simulink model "play"  (R2024a)
settings: Solver=ode1  StartTime=0.0  StopTime=inf  FixedStep=1/10  RelTol=1e-3  EnableMultiTasking=on
undefined symbols (not defined in the file): HIL, Host
libraries: quarc_library x8, simulink_extras x1, simulink x1
settings Model: Creator=msaravanan  LastModifiedBy=msaravanan
settings SolverCC: PositivePriorityOrder=on
settings RTWCC: Description=QUARC Win64 Target Using Toolchain  SystemTargetFile=quarc_win64.tlc  Toolchain=QUARC win64 | nmake (64-bit Windows)  BuildConfiguration=Faster Runs
settings STFCustomTargetCC: ConcurrentExecutionCompliant=on  SystemTargetFile=quarc_win64.tlc
settings GRTTargetCC: ParMdlRefBuildCompliant=off  CompOptLevelCompliant=off  CombineOutputUpdateFcns=off  MatFileLogging=off  CPPClassGenCompliant=off  GRTInterface=on  ExtMode=on  ExtModeMexFile=quarc_comm

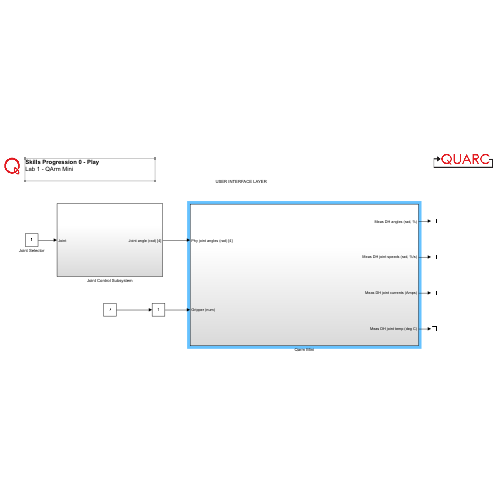
[thumbnail: Simulink's stored preview of the top-level diagram]
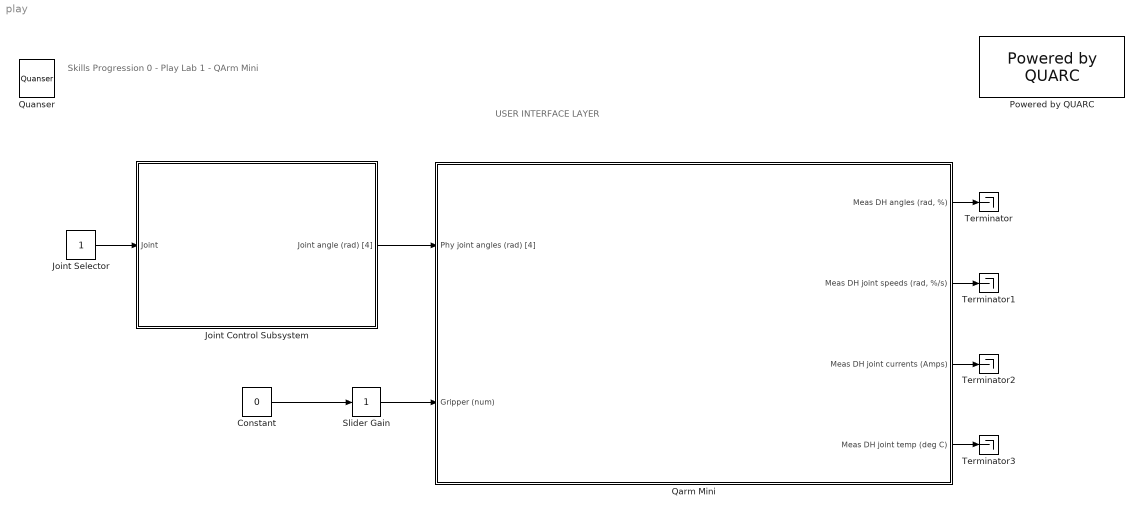
== system play ==
  note: USER INTERFACE LAYER
  note: Skills Progression 0 - Play
      | Lab 1 - QArm Mini
  Constant : Constant  Value=0
  Joint Control Subsystem : Subsystem
  Joint Selector : Constant
  Powered by QUARC : quarc_library/Logos/Powered by QUARC
  Qarm Mini : Subsystem
  Quanser : quarc_library/Logos/Quanser
  Slider Gain : simulink/Math Operations/Slider Gain  gain=1  low=0  high=2
  Terminator{,1..3} (4 alike) : Terminator
  wires:
  Slider Gain/1 -> Qarm Mini/2(Gripper (num))
  Qarm Mini/1("Meas DH angles (rad, %)") -> Terminator/1
  Qarm Mini/2("Meas DH joint speeds (rad, %/s)") -> Terminator1/1
  Qarm Mini/3(Meas DH joint currents (Amps)) -> Terminator2/1
  Qarm Mini/4(Meas DH joint temp (deg C)) -> Terminator3/1
  Joint Selector/1 -> Joint Control Subsystem/1(Joint)
  Constant/1 -> Slider Gain/1
  Joint Control Subsystem/1(Joint angle (rad) [4]) -> Qarm Mini/1(Phy joint angles (rad) [4])

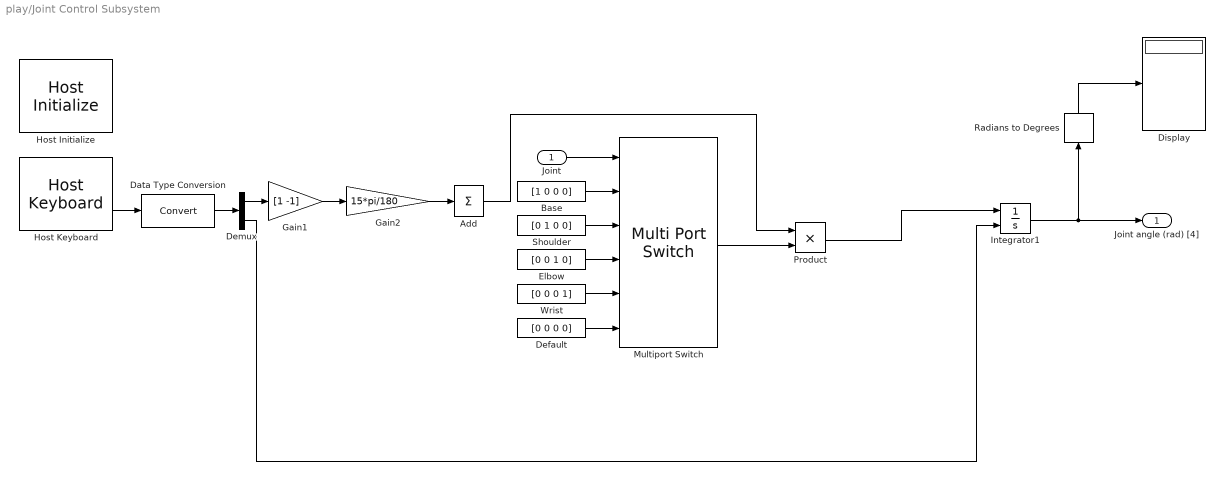
== system play/Joint Control Subsystem ==
  Joint : Inport
  Add : Sum  Inputs=1
  Base : Constant  Value=[1 0 0 0]
  Data Type Conversion : DataTypeConversion  SaturateOnIntegerOverflow=off  RndMeth=Floor
  Default : Constant  Value=[0 0 0 0]
  Demux : Demux  Outputs=2
  Display : Display
  Elbow : Constant  Value=[0 0 1 0]
  Gain1 : Gain  Gain=[1 -1]
  Gain2 : Gain  Gain=15*pi/180
  Host Initialize : quarc_library/Devices/Peripherals/Host/Host Initialize  object_name=Host-1  uri_source=Use external mode communications  uri=tcpip://localhost:18001  send_buffer_size=1000  receive_buffer_size=1000  thread_priority=0  run_client=on  use_window=off  window_position=[]  sample_time=qc_get_step_size  active=on
      settings: SourceProductName=QUARC Targets
  Host Keyboard : quarc_library/Devices/Peripherals/Host/Host Keyboard  object_name=Host-1  virtual_key="[38  40  32]"  sample_time=qc_get_step_size  enabled=on  debug_mode=off
      settings: SourceProductName=QUARC Targets
  Integrator1 : Integrator  ExternalReset=rising  LimitOutput=on  UpperSaturationLimit=[5*pi/4, pi/2, pi/2, pi/4]  LowerSaturationLimit=[-pi/2. -pi/2, -pi/4, -pi/2]
  Multiport Switch : MultiPortSwitch  Inputs=5  DiagnosticForDefault=Warning  SaturateOnIntegerOverflow=off  InputSameDT=off
  Product : Product
  Radians to Degrees : simulink_extras/Transformations/Radians to Degrees
  Shoulder : Constant  Value=[0 1 0 0]
  Wrist : Constant  Value=[0 0 0 1]
  Joint angle (rad) [4] : Outport
  wires:
  Host Keyboard/2 -> Data Type Conversion/1
  Demux/1 -> Gain1/1
  Data Type Conversion/1 -> Demux/1
  Gain2/1 -> Add/1
  Gain1/1 -> Gain2/1
  Default/1 -> Multiport Switch/6
  Joint/1 -> Multiport Switch/1
  Add/1 -> Product/1
  Multiport Switch/1 -> Product/2
  Shoulder/1 -> Multiport Switch/3
  Elbow/1 -> Multiport Switch/4
  Wrist/1 -> Multiport Switch/5
  Product/1 -> Integrator1/1
  Base/1 -> Multiport Switch/2
  Radians to Degrees/1 -> Display/1
  Demux/2 -> Integrator1/2
  Integrator1/1 -> Joint angle (rad) [4]/1, Radians to Degrees/1

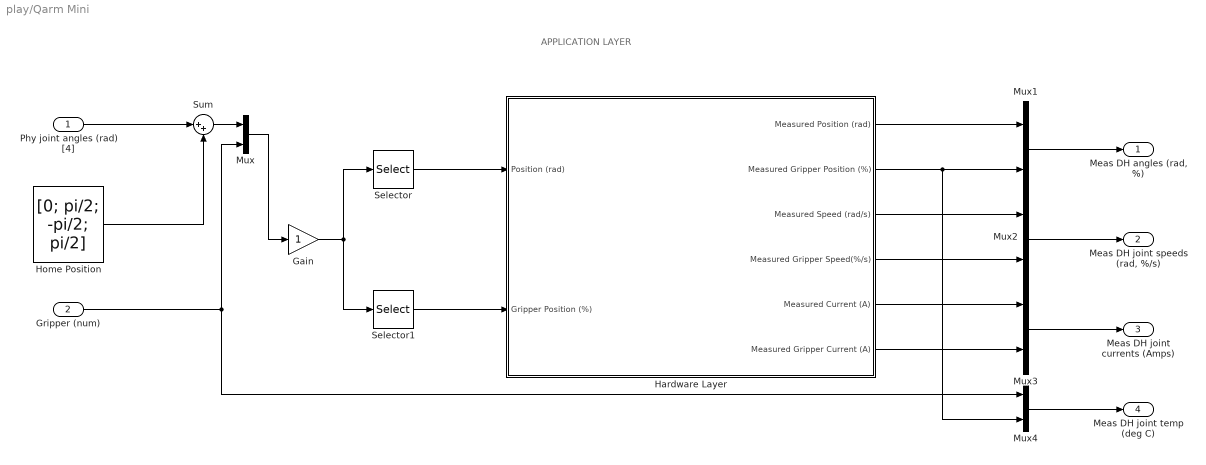
== system play/Qarm Mini ==
  note: APPLICATION LAYER
  Phy joint angles (rad) [4] : Inport
  Gripper (num) : Inport  Port=2
  Gain : Gain
  Hardware Layer : Subsystem
  Home Position : Constant  Value=[0; pi/2; -pi/2; pi/2]  VectorParams1D=off
  Mux{,1..4} (5 alike) : Mux  Inputs=2
  Selector : Selector  InputPortWidth=5  IndexOptions=Index vector (dialog)  Indices=1:4  OutputSizes=1
  Selector1 : Selector  InputPortWidth=5  IndexOptions=Index vector (dialog)  Indices=5  OutputSizes=1
  Sum : Sum  Inputs=|++
  "Meas DH angles (rad, %)" : Outport
  "Meas DH joint speeds (rad, %/s)" : Outport  Port=2
  Meas DH joint currents (Amps) : Outport  Port=3
  Meas DH joint temp (deg C) : Outport  Port=4
  wires:
  Phy joint angles (rad) [4]/1 -> Sum/1
  Home Position/1 -> Sum/2
  Sum/1 -> Mux/1
  Gripper (num)/1 -> Mux/2, Mux4/1
  Mux/1 -> Gain/1
  Gain/1 -> Selector1/1, Selector/1
  Hardware Layer/1(Measured Position (rad)) -> Mux1/1
  Hardware Layer/2(Measured Gripper Position (%)) -> Mux4/2, Mux1/2
  Hardware Layer/3(Measured Speed (rad/s)) -> Mux2/1
  Hardware Layer/4(Measured Gripper Speed(%/s)) -> Mux2/2
  Hardware Layer/5(Measured Current (A)) -> Mux3/1
  Hardware Layer/6(Measured Gripper Current (A)) -> Mux3/2
  Mux4/1 -> Meas DH joint temp (deg C)/1
  Mux3/1 -> Meas DH joint currents (Amps)/1
  Mux2/1 -> "Meas DH joint speeds (rad, %/s)"/1
  Mux1/1 -> "Meas DH angles (rad, %)"/1
  Selector/1 -> Hardware Layer/1(Position (rad))
  Selector1/1 -> Hardware Layer/2(Gripper Position (%))

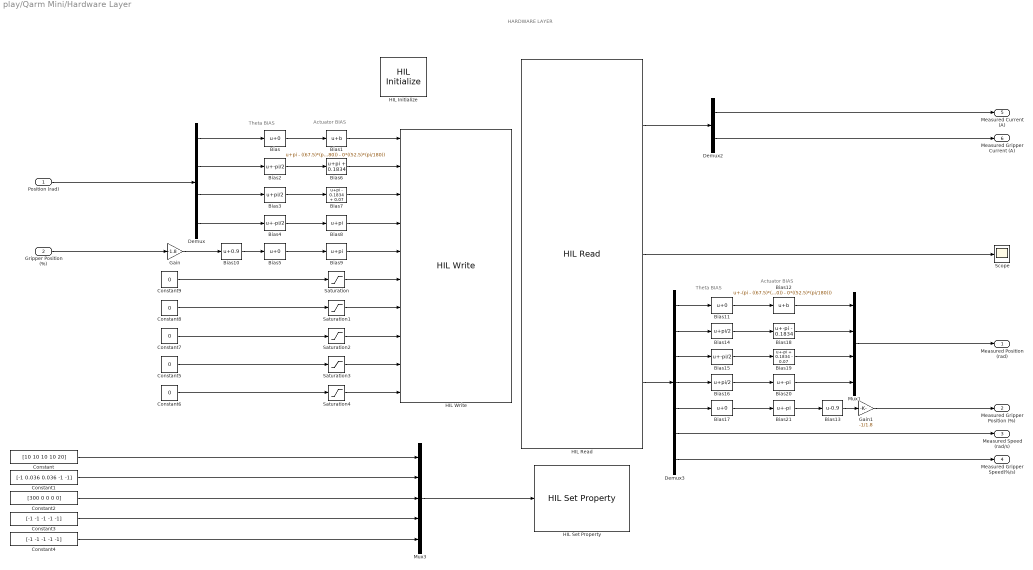
== system play/Qarm Mini/Hardware Layer ==
  note: HARDWARE LAYER
  note: Actuator BIAS
  note: Theta BIAS
  note: Actuator BIAS
  note: Theta BIAS
  Position (rad) : Inport
  Gripper Position (%) : Inport  Port=2
  Bias{,5,11,17} (4 alike) : Bias  SaturateOnIntegerOverflow=off
  Bias1 : Bias  Bias=pi - ((67.5)*(pi/180)) - 0*((52.5)*(pi/180))  SaturateOnIntegerOverflow=off
  Bias10 : Bias  Bias=0.9  SaturateOnIntegerOverflow=off
  Bias12 : Bias  Bias=-(pi - ((67.5)*(pi/180)) - 0*((52.5)*(pi/180)))  SaturateOnIntegerOverflow=off
  Bias13 : Bias  Bias=-0.9  SaturateOnIntegerOverflow=off
  Bias14 : Bias  Bias=pi/2  SaturateOnIntegerOverflow=off
  Bias15 : Bias  Bias=-pi/2  SaturateOnIntegerOverflow=off
  Bias16 : Bias  Bias=pi/2  SaturateOnIntegerOverflow=off
  Bias18 : Bias  Bias="-pi -  0.1834"  SaturateOnIntegerOverflow=off
  Bias19 : Bias  Bias="-pi +  0.1834 - 0.07"  SaturateOnIntegerOverflow=off
  Bias2 : Bias  Bias=-pi/2  SaturateOnIntegerOverflow=off
  Bias20 : Bias  Bias=-pi  SaturateOnIntegerOverflow=off
  Bias21 : Bias  Bias=-pi  SaturateOnIntegerOverflow=off
  Bias3 : Bias  Bias=pi/2  SaturateOnIntegerOverflow=off
  Bias4 : Bias  Bias=-pi/2  SaturateOnIntegerOverflow=off
  Bias6 : Bias  Bias=pi + 0.1834  SaturateOnIntegerOverflow=off
  Bias7 : Bias  Bias="pi -  0.1834 + 0.07"  SaturateOnIntegerOverflow=off
  Bias8 : Bias  Bias=pi  SaturateOnIntegerOverflow=off
  Bias9 : Bias  Bias=pi  SaturateOnIntegerOverflow=off
  Constant : Constant  Value=[10 10 10 10 20]
  Constant1 : Constant  Value=[-1 0.036 0.036 -1 -1]
  Constant2 : Constant  Value=[300 0 0 0 0]
  Constant3 : Constant  Value=[-1 -1 -1 -1 -1]
  Constant4 : Constant  Value=[-1 -1 -1 -1 -1]
  Constant{5..9} (5 alike) : Constant  Value=0
  Demux : Demux
  Demux2 : Demux  Outputs=[4 1]
  Demux3 : Demux  Outputs=[1 1 1 1 1 4 1]
  Gain : Gain  Gain=-1.8
  Gain1 : Gain  Gain=-1/1.8
  HIL Initialize : quarc_library/Data Acquisition/Generic/Configuration/HIL Initialize  object_name=HIL-2  board_type=qarm_mini  board_number=4  board_options=j0_mode=0;j1_mode=0;j2_mode=0;j3_mode=0;gripper_mode=0;j0_profile_velocity=6.2832;j0_profile_acceleration=6.2832;j1_profile_velocity=6.2832;j1_profile_acceleration=6.2832;j2_profile_velocity=6.2832;j2_profile_acceleration=6.2832;j3_profile_velocity=6.2832;j3_profile_acceleration=6.2832;gripper_profile_velocity=6.2832;gripper_profile_acceleration=6.2832;  exclusive=off  active=on  hardware_clocks=[]  clock_modes=[]  initial_clock_frequencies=[]  set_clock_params_at_start=off  set_clock_params_at_switch_in=off  set_clock_frequencies_at_start=off  set_clock_frequencies_at_switch_in=off  analog_input_channels=[0:4]  analog_input_configurations=[]  analog_input_maximums=[100 3.21 3.21 3.21 100]  analog_input_minimums=[-100 -3.21 -3.21 -3.21 -100]  set_analog_input_params_at_start=off  set_analog_input_params_at_switch_in=off  analog_output_channels=[]  analog_output_maximums=[]  analog_output_minimums=[]  initial_analog_outputs=[]  final_analog_outputs=[]  watchdog_analog_outputs=[]  set_analog_output_params_at_start=off  set_analog_output_params_at_switch_in=off  set_analog_outputs_at_start=off  set_analog_outputs_at_switch_in=off  set_analog_outputs_at_terminate=off  set_analog_outputs_at_switch_out=off  set_analog_outputs_on_watchdog=off  digital_input_channels=[]  digital_output_channels=[]  digital_output_configuration=[]  initial_digital_outputs=[]  final_digital_outputs=[]  watchdog_digital_outputs=[]  set_digital_output_params_at_start=off  set_digital_output_params_at_switch_in=off  set_digital_outputs_at_start=off  set_digital_outputs_at_switch_in=off  set_digital_outputs_at_terminate=off  set_digital_outputs_at_switch_out=off  set_digital_outputs_on_watchdog=off  encoder_channels=[]  quadrature=[]  encoder_filter_frequency=[]  initial_encoder_counts=[]  set_encoder_params_at_start=off  set_encoder_params_at_switch_in=off  set_encoder_counts_at_start=off  set_encoder_counts_at_switch_in=off  pwm_channels=[]  pwm_modes=[]  pwm_frequency=[]  pwm_configuration=[]  pwm_alignment=[]  pwm_polarity=[]  pwm_leading_deadband=[]  pwm_trailing_deadband=[]  initial_pwm_outputs=[]  final_pwm_outputs=[]  watchdog_pwm_outputs=[]  set_pwm_params_at_start=off  set_pwm_params_at_switch_in=off  set_pwm_outputs_at_start=off  set_pwm_outputs_at_switch_in=off  set_pwm_outputs_at_terminate=off  set_pwm_outputs_at_switch_out=off  set_pwm_outputs_on_watchdog=off  other_output_channels=[]  initial_other_outputs=[]  final_other_outputs=[]  watchdog_other_outputs=[]  set_other_outputs_at_start=off  set_other_outputs_at_switch_in=off  set_other_outputs_at_terminate=off  set_other_outputs_at_switch_out=off  set_other_outputs_on_watchdog=off
  HIL Read : quarc_library/Data Acquisition/Generic/Immediate I//O/HIL Read  object_name=HIL-2  analog_channels=[0:4]  encoder_channels=[]  digital_channels=[0:24]  other_channels=[1000:1004 3000:3004]  sample_time=qc_get_step_size  active=on  vector_output=on  data_type_mode=Inherit via back propagation  encoder_data_type=double  digital_data_type=boolean
  HIL Set Property : quarc_library/Data Acquisition/Generic/Configuration/HIL Set Property  object_name=HIL-2  property_type=2  property_codes=[128:152]  property_source=2  property_value_num=0  set_at_start=on  sample_time=-1  active=off
      settings: AttributesFormatString=(%<object_name>)  SourceProductName=QUARC Targets
  HIL Write : quarc_library/Data Acquisition/Generic/Immediate I//O/HIL Write  object_name=HIL-2  analog_channels=[]  pwm_channels=[]  digital_channels=[]  other_channels=[1000:1004 11000:11004]  sample_time=-1  active=off  vector_input=off
  Mux1 : Mux
  Mux3 : Mux  Inputs=5
  Saturation{,1..4} (5 alike) : Saturate
  Scope : Scope
  Measured Position (rad) : Outport
  Measured Gripper Position (%) : Outport  Port=2
  Measured Speed (rad/s) : Outport  Port=3
  Measured Gripper Speed(%/s) : Outport  Port=4
  Measured Current (A) : Outport  Port=5
  Measured Gripper Current (A) : Outport  Port=6
  wires:
  Position (rad)/1 -> Demux/1
  Demux/1 -> Bias/1
  Demux/2 -> Bias2/1
  Demux/3 -> Bias3/1
  Demux/4 -> Bias4/1
  Bias/1 -> Bias1/1
  Bias1/1 -> HIL Write/1
  Bias2/1 -> Bias6/1
  Bias3/1 -> Bias7/1
  Bias7/1 -> HIL Write/3
  Bias4/1 -> Bias8/1
  Bias8/1 -> HIL Write/4
  Bias5/1 -> Bias9/1
  Bias9/1 -> HIL Write/5
  Gripper Position (%)/1 -> Gain/1
  Gain/1 -> Bias10/1
  Bias10/1 -> Bias5/1
  Constant9/1 -> Saturation/1
  Constant8/1 -> Saturation1/1
  Constant7/1 -> Saturation2/1
  Constant5/1 -> Saturation3/1
  Constant6/1 -> Saturation4/1
  Saturation/1 -> HIL Write/6
  Saturation1/1 -> HIL Write/7
  Saturation2/1 -> HIL Write/8
  Saturation3/1 -> HIL Write/9
  Saturation4/1 -> HIL Write/10
  Bias14/1 -> Bias18/1
  Bias15/1 -> Bias19/1
  Bias17/1 -> Bias21/1
  Bias11/1 -> Bias12/1
  Bias16/1 -> Bias20/1
  Bias21/1 -> Bias13/1
  Bias13/1 -> Gain1/1
  Gain1/1 -> Measured Gripper Position (%)/1
  Bias12/1 -> Mux1/1
  Bias18/1 -> Mux1/2
  Bias19/1 -> Mux1/3
  Bias20/1 -> Mux1/4
  Mux1/1 -> Measured Position (rad)/1
  Demux3/6 -> Measured Speed (rad/s)/1
  Constant/1 -> Mux3/1
  Constant1/1 -> Mux3/2
  Constant2/1 -> Mux3/3
  Constant3/1 -> Mux3/4
  Constant4/1 -> Mux3/5
  Mux3/1 -> HIL Set Property/1
  Demux2/2 -> Measured Gripper Current (A)/1
  HIL Read/1 -> Demux2/1
  Demux2/1 -> Measured Current (A)/1
  Demux3/1 -> Bias11/1
  Demux3/2 -> Bias14/1
  Demux3/3 -> Bias15/1
  Demux3/4 -> Bias16/1
  Demux3/5 -> Bias17/1
  Demux3/7 -> Measured Gripper Speed(%/s)/1
  HIL Read/3 -> Demux3/1
  HIL Read/2 -> Scope/1
  Bias6/1 -> HIL Write/2
